simulink model "kundur_cvs_v3_discrete"  (R2025b)
settings: Solver=FixedStepAuto  StartTime=0.0  StopTime=0.5  FixedStep=50e-6  RelTol=1e-3
values from neighbouring files (symbols this model uses):
  delta0_1 = 0.294539737007    [kundur_cvs_v3_discrete_runtime.mat]    (also in kundur_cvs_v3_runtime.mat)
  delta0_2 = 0.0944024626245    [kundur_cvs_v3_discrete_runtime.mat]    (also in kundur_cvs_v3_runtime.mat)
  delta0_3 = 0.25103283995    [kundur_cvs_v3_discrete_runtime.mat]    (also in kundur_cvs_v3_runtime.mat)
  delta0_4 = 0.0812572055811    [kundur_cvs_v3_discrete_runtime.mat]    (also in kundur_cvs_v3_runtime.mat)
  deltaG0_1 = 0.522124293082    [kundur_cvs_v3_discrete_runtime.mat]    (also in kundur_cvs_v3_runtime.mat)
  deltaG0_2 = 0.476153951225    [kundur_cvs_v3_discrete_runtime.mat]    (also in kundur_cvs_v3_runtime.mat)
  deltaG0_3 = 0.293879837027    [kundur_cvs_v3_discrete_runtime.mat]    (also in kundur_cvs_v3_runtime.mat)
  Dg_1 = 5    [kundur_cvs_v3_discrete_runtime.mat]    (also in kundur_cvs_v3_runtime.mat)
  Dg_2 = 5    [kundur_cvs_v3_discrete_runtime.mat]    (also in kundur_cvs_v3_runtime.mat)
  Dg_3 = 5    [kundur_cvs_v3_discrete_runtime.mat]    (also in kundur_cvs_v3_runtime.mat)
  LoadStep_amp_bus14 = 248000000    [kundur_cvs_v3_discrete_runtime.mat]    (also in kundur_cvs_v3_runtime.mat)
  LoadStep_amp_bus15 = 0    [kundur_cvs_v3_discrete_runtime.mat]    (also in kundur_cvs_v3_runtime.mat)
  LoadStep_t_bus14 = 5    [kundur_cvs_v3_discrete_runtime.mat]    (also in kundur_cvs_v3_runtime.mat)
  LoadStep_t_bus15 = 5    [kundur_cvs_v3_discrete_runtime.mat]    (also in kundur_cvs_v3_runtime.mat)
  Mg_1 = 13    [kundur_cvs_v3_discrete_runtime.mat]    (also in kundur_cvs_v3_runtime.mat)
  Mg_2 = 13    [kundur_cvs_v3_discrete_runtime.mat]    (also in kundur_cvs_v3_runtime.mat)
  Mg_3 = 12.35    [kundur_cvs_v3_discrete_runtime.mat]    (also in kundur_cvs_v3_runtime.mat)
  Pe_scale = 1e-08    [kundur_cvs_runtime.mat]    (also in kundur_cvs_v3_discrete_runtime.mat; kundur_cvs_v3_runtime.mat)
  Pm_1 = 0.250224865012    [kundur_cvs_v3_discrete_runtime.mat]    (also in kundur_cvs_v3_runtime.mat)
  Pm_2 = 0.250224865012    [kundur_cvs_v3_discrete_runtime.mat]    (also in kundur_cvs_v3_runtime.mat)
  Pm_3 = 0.250224865012    [kundur_cvs_v3_discrete_runtime.mat]    (also in kundur_cvs_v3_runtime.mat)
  Pm_4 = 0.250224865012    [kundur_cvs_v3_discrete_runtime.mat]    (also in kundur_cvs_v3_runtime.mat)
  Pmg_1 = 7.00000000011    [kundur_cvs_v3_discrete_runtime.mat]    (also in kundur_cvs_v3_runtime.mat)
  Pmg_2 = 7    [kundur_cvs_v3_discrete_runtime.mat]    (also in kundur_cvs_v3_runtime.mat)
  Pmg_3 = 7.19    [kundur_cvs_v3_discrete_runtime.mat]    (also in kundur_cvs_v3_runtime.mat)
  PmgStep_amp_1 = 0    [kundur_cvs_v3_discrete_runtime.mat]    (also in kundur_cvs_v3_runtime.mat)
  PmgStep_amp_2 = 0    [kundur_cvs_v3_discrete_runtime.mat]    (also in kundur_cvs_v3_runtime.mat)
  PmgStep_amp_3 = 0    [kundur_cvs_v3_discrete_runtime.mat]    (also in kundur_cvs_v3_runtime.mat)
  PmgStep_t_1 = 5    [kundur_cvs_v3_discrete_runtime.mat]    (also in kundur_cvs_v3_runtime.mat)
  PmgStep_t_2 = 5    [kundur_cvs_v3_discrete_runtime.mat]    (also in kundur_cvs_v3_runtime.mat)
  PmgStep_t_3 = 5    [kundur_cvs_v3_discrete_runtime.mat]    (also in kundur_cvs_v3_runtime.mat)
  Rg_1 = 0.05    [kundur_cvs_v3_discrete_runtime.mat]    (also in kundur_cvs_v3_runtime.mat)
  Rg_2 = 0.05    [kundur_cvs_v3_discrete_runtime.mat]    (also in kundur_cvs_v3_runtime.mat)
  Rg_3 = 0.05    [kundur_cvs_v3_discrete_runtime.mat]    (also in kundur_cvs_v3_runtime.mat)
  SGScale_1 = 0.111111111111    [kundur_cvs_v3_discrete_runtime.mat]    (also in kundur_cvs_v3_runtime.mat)
  SGScale_2 = 0.111111111111    [kundur_cvs_v3_discrete_runtime.mat]    (also in kundur_cvs_v3_runtime.mat)
  SGScale_3 = 0.111111111111    [kundur_cvs_v3_discrete_runtime.mat]    (also in kundur_cvs_v3_runtime.mat)
  VemfG_1 = 266775.927939    [kundur_cvs_v3_discrete_runtime.mat]    (also in kundur_cvs_v3_runtime.mat)
  VemfG_2 = 255963.649879    [kundur_cvs_v3_discrete_runtime.mat]    (also in kundur_cvs_v3_runtime.mat)
  VemfG_3 = 266432.593136    [kundur_cvs_v3_discrete_runtime.mat]    (also in kundur_cvs_v3_runtime.mat)
  Vmag_1 = 230000    [kundur_cvs_runtime.mat]    (also in kundur_cvs_v3_discrete_runtime.mat = 201813.659575; kundur_cvs_v3_runtime.mat = 201813.659575)
  Vmag_2 = 230000    [kundur_cvs_runtime.mat]    (also in kundur_cvs_v3_discrete_runtime.mat = 232642.850172; kundur_cvs_v3_runtime.mat = 232642.850172)
  Vmag_3 = 230000    [kundur_cvs_runtime.mat]    (also in kundur_cvs_v3_discrete_runtime.mat = 178957.562058; kundur_cvs_v3_runtime.mat = 178957.562058)
  Vmag_4 = 230000    [kundur_cvs_runtime.mat]    (also in kundur_cvs_v3_discrete_runtime.mat = 226974.072481; kundur_cvs_v3_runtime.mat = 226974.072481)
  VSGScale_1 = 0.5    [kundur_cvs_v3_discrete_runtime.mat]    (also in kundur_cvs_v3_runtime.mat)
  VSGScale_2 = 0.5    [kundur_cvs_v3_discrete_runtime.mat]    (also in kundur_cvs_v3_runtime.mat)
  VSGScale_3 = 0.5    [kundur_cvs_v3_discrete_runtime.mat]    (also in kundur_cvs_v3_runtime.mat)
  VSGScale_4 = 0.5    [kundur_cvs_v3_discrete_runtime.mat]    (also in kundur_cvs_v3_runtime.mat)
  WindAmp_1 = 1    [kundur_cvs_v3_discrete_runtime.mat]    (also in kundur_cvs_v3_runtime.mat)
  WindAmp_2 = 1    [kundur_cvs_v3_discrete_runtime.mat]    (also in kundur_cvs_v3_runtime.mat)
  wn_const = 314.159265359    [kundur_cvs_runtime.mat]    (also in kundur_cvs_v3_discrete_runtime.mat; kundur_cvs_v3_runtime.mat)
  Wphase_1 = 0.0648179941055    [kundur_cvs_v3_discrete_runtime.mat]    (also in kundur_cvs_v3_runtime.mat)
  Wphase_2 = 0.0587091014116    [kundur_cvs_v3_discrete_runtime.mat]    (also in kundur_cvs_v3_runtime.mat)
  WVmag_1 = 230000    [kundur_cvs_v3_discrete_runtime.mat]    (also in kundur_cvs_v3_runtime.mat)
  WVmag_2 = 230000    [kundur_cvs_v3_discrete_runtime.mat]    (also in kundur_cvs_v3_runtime.mat)
undefined symbols (not defined in the file or in its folder): D_1, D_2, D_3, D_4, M_1, M_2, M_3, M_4, Pm_step_amp_1, Pm_step_amp_2, Pm_step_amp_3, Pm_step_amp_4, Pm_step_t_1, Pm_step_t_2, Pm_step_t_3, Pm_step_t_4
libraries: spsControlledVoltageSourceLib x21, spsSeriesRLCBranchLib x21, spsThreePhasePISectionLineLib x19, spsGroundLib x7, spsThreePhaseVIMeasurementLib x7, spsThreePhaseSeriesRLCLoadLib x6, spsThreePhaseBreakerLib x2, spsThreePhaseSourceLib x2, spspowerguiLib x1
settings Model: Creator=27443  LastModifiedBy=27443

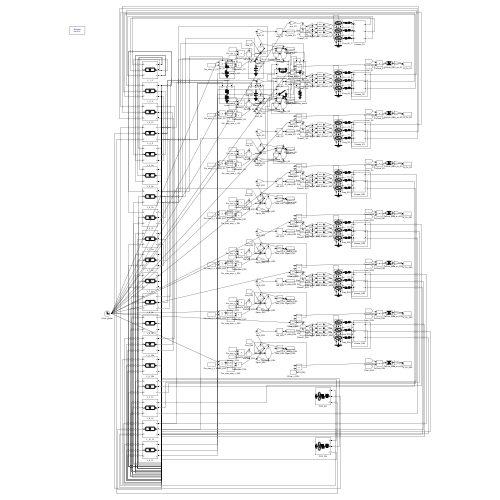
[thumbnail: Simulink's stored preview of the top-level diagram]
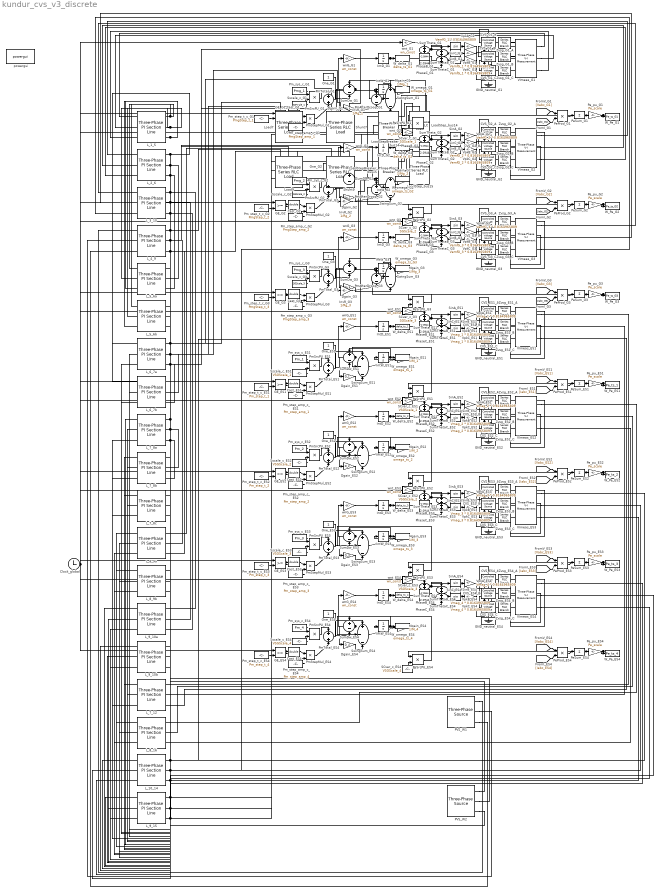
== system kundur_cvs_v3_discrete ==
  CVS_ES1_A : spsControlledVoltageSourceLib/Controlled Voltage Source  Initialize=on  Source_Type=AC  Amplitude=0  Phase=0  Frequency=0  Measurements=None
  CVS_ES1_B : spsControlledVoltageSourceLib/Controlled Voltage Source  Initialize=on  Source_Type=AC  Amplitude=0  Phase=0  Frequency=0  Measurements=None
  CVS_ES1_C : spsControlledVoltageSourceLib/Controlled Voltage Source  Initialize=on  Source_Type=AC  Amplitude=0  Phase=0  Frequency=0  Measurements=None
  CVS_ES2_A : spsControlledVoltageSourceLib/Controlled Voltage Source  Initialize=on  Source_Type=AC  Amplitude=0  Phase=0  Frequency=0  Measurements=None
  CVS_ES2_B : spsControlledVoltageSourceLib/Controlled Voltage Source  Initialize=on  Source_Type=AC  Amplitude=0  Phase=0  Frequency=0  Measurements=None
  CVS_ES2_C : spsControlledVoltageSourceLib/Controlled Voltage Source  Initialize=on  Source_Type=AC  Amplitude=0  Phase=0  Frequency=0  Measurements=None
  CVS_ES3_A : spsControlledVoltageSourceLib/Controlled Voltage Source  Initialize=on  Source_Type=AC  Amplitude=0  Phase=0  Frequency=0  Measurements=None
  CVS_ES3_B : spsControlledVoltageSourceLib/Controlled Voltage Source  Initialize=on  Source_Type=AC  Amplitude=0  Phase=0  Frequency=0  Measurements=None
  CVS_ES3_C : spsControlledVoltageSourceLib/Controlled Voltage Source  Initialize=on  Source_Type=AC  Amplitude=0  Phase=0  Frequency=0  Measurements=None
  CVS_ES4_A : spsControlledVoltageSourceLib/Controlled Voltage Source  Initialize=on  Source_Type=AC  Amplitude=0  Phase=0  Frequency=0  Measurements=None
  CVS_ES4_B : spsControlledVoltageSourceLib/Controlled Voltage Source  Initialize=on  Source_Type=AC  Amplitude=0  Phase=0  Frequency=0  Measurements=None
  CVS_ES4_C : spsControlledVoltageSourceLib/Controlled Voltage Source  Initialize=on  Source_Type=AC  Amplitude=0  Phase=0  Frequency=0  Measurements=None
  CVS_G1_A : spsControlledVoltageSourceLib/Controlled Voltage Source  Initialize=on  Source_Type=AC  Amplitude=0  Phase=0  Frequency=0  Measurements=None
  CVS_G1_B : spsControlledVoltageSourceLib/Controlled Voltage Source  Initialize=on  Source_Type=AC  Amplitude=0  Phase=0  Frequency=0  Measurements=None
  CVS_G1_C : spsControlledVoltageSourceLib/Controlled Voltage Source  Initialize=on  Source_Type=AC  Amplitude=0  Phase=0  Frequency=0  Measurements=None
  CVS_G2_A : spsControlledVoltageSourceLib/Controlled Voltage Source  Initialize=on  Source_Type=AC  Amplitude=0  Phase=0  Frequency=0  Measurements=None
  CVS_G2_B : spsControlledVoltageSourceLib/Controlled Voltage Source  Initialize=on  Source_Type=AC  Amplitude=0  Phase=0  Frequency=0  Measurements=None
  CVS_G2_C : spsControlledVoltageSourceLib/Controlled Voltage Source  Initialize=on  Source_Type=AC  Amplitude=0  Phase=0  Frequency=0  Measurements=None
  CVS_G3_A : spsControlledVoltageSourceLib/Controlled Voltage Source  Initialize=on  Source_Type=AC  Amplitude=0  Phase=0  Frequency=0  Measurements=None
  CVS_G3_B : spsControlledVoltageSourceLib/Controlled Voltage Source  Initialize=on  Source_Type=AC  Amplitude=0  Phase=0  Frequency=0  Measurements=None
  CVS_G3_C : spsControlledVoltageSourceLib/Controlled Voltage Source  Initialize=on  Source_Type=AC  Amplitude=0  Phase=0  Frequency=0  Measurements=None
  Cast_ES{1..4} (4 alike) : DataTypeConversion  OutDataTypeStr=double  SaturateOnIntegerOverflow=off  RndMeth=Floor
  Cast_G1 : DataTypeConversion  OutDataTypeStr=double  SaturateOnIntegerOverflow=off  RndMeth=Floor
  Cast_G2 : DataTypeConversion  OutDataTypeStr=double  SaturateOnIntegerOverflow=off  RndMeth=Floor
  Cast_G3 : DataTypeConversion  OutDataTypeStr=double  SaturateOnIntegerOverflow=off  RndMeth=Floor
  Clock_global : Clock
  Dgain_ES1 : Gain  Gain=D_1
  Dgain_ES2 : Gain  Gain=D_2
  Dgain_ES3 : Gain  Gain=D_3
  Dgain_ES4 : Gain  Gain=D_4
  Dgain_G1 : Gain  Gain=Dg_1
  Dgain_G2 : Gain  Gain=Dg_2
  Dgain_G3 : Gain  Gain=Dg_3
  GE_ES{1..4} (4 alike) : RelationalOperator  OutDataTypeStr=boolean  RndMeth=Simplest  InputSameDT=off
  GE_G1 : RelationalOperator  OutDataTypeStr=boolean  RndMeth=Simplest  InputSameDT=off
  GE_G2 : RelationalOperator  OutDataTypeStr=boolean  RndMeth=Simplest  InputSameDT=off
  GE_G3 : RelationalOperator  OutDataTypeStr=boolean  RndMeth=Simplest  InputSameDT=off
  GND_neutral_ES{1..4} (4 alike) : spsGroundLib/Ground  LConnTagsString=a
  GND_neutral_G1 : spsGroundLib/Ground  LConnTagsString=a
  GND_neutral_G2 : spsGroundLib/Ground  LConnTagsString=a
  GND_neutral_G3 : spsGroundLib/Ground  LConnTagsString=a
  IntD_ES1 : Integrator  InitialCondition=delta0_1
  IntD_ES2 : Integrator  InitialCondition=delta0_2
  IntD_ES3 : Integrator  InitialCondition=delta0_3
  IntD_ES4 : Integrator  InitialCondition=delta0_4
  IntD_G1 : Integrator  InitialCondition=deltaG0_1
  IntD_G2 : Integrator  InitialCondition=deltaG0_2
  IntD_G3 : Integrator  InitialCondition=deltaG0_3
  IntW_ES{1..4} (4 alike) : Integrator  InitialCondition=1
  IntW_G1 : Integrator  InitialCondition=1
  IntW_G2 : Integrator  InitialCondition=1
  IntW_G3 : Integrator  InitialCondition=1
  InvR_G1 : Gain  Gain=1/Rg_1
  InvR_G2 : Gain  Gain=1/Rg_2
  InvR_G3 : Gain  Gain=1/Rg_3
  L_10_14 : spsThreePhasePISectionLineLib/Three-Phase PI Section Line  LConnTagsString=a|b|c  RConnTagsString=A|B|C  Length=1  Frequency=50  Resistances=[0.01 0.03]  Inductances=[0.0005 0.0015]  Capacitances=[2.55102040816327e-08 1.53061224489796e-08]
  L_1_5 : spsThreePhasePISectionLineLib/Three-Phase PI Section Line  LConnTagsString=a|b|c  RConnTagsString=A|B|C  Length=5  Frequency=50  Resistances=[0.053 0.159]  Inductances=[0.00141 0.00423]  Capacitances=[9.04617166015342e-09 5.42770299609205e-09]
  L_2_6 : spsThreePhasePISectionLineLib/Three-Phase PI Section Line  LConnTagsString=a|b|c  RConnTagsString=A|B|C  Length=5  Frequency=50  Resistances=[0.053 0.159]  Inductances=[0.00141 0.00423]  Capacitances=[9.04617166015342e-09 5.42770299609205e-09]
  L_3_10 : spsThreePhasePISectionLineLib/Three-Phase PI Section Line  LConnTagsString=a|b|c  RConnTagsString=A|B|C  Length=5  Frequency=50  Resistances=[0.053 0.159]  Inductances=[0.00141 0.00423]  Capacitances=[9.04617166015342e-09 5.42770299609205e-09]
  L_4_9 : spsThreePhasePISectionLineLib/Three-Phase PI Section Line  LConnTagsString=a|b|c  RConnTagsString=A|B|C  Length=5  Frequency=50  Resistances=[0.053 0.159]  Inductances=[0.00141 0.00423]  Capacitances=[9.04617166015342e-09 5.42770299609205e-09]
  L_5_6a : spsThreePhasePISectionLineLib/Three-Phase PI Section Line  LConnTagsString=a|b|c  RConnTagsString=A|B|C  Length=25  Frequency=50  Resistances=[0.053 0.159]  Inductances=[0.00141 0.00423]  Capacitances=[9.04617166015342e-09 5.42770299609205e-09]
  L_5_6b : spsThreePhasePISectionLineLib/Three-Phase PI Section Line  LConnTagsString=a|b|c  RConnTagsString=A|B|C  Length=25  Frequency=50  Resistances=[0.053 0.159]  Inductances=[0.00141 0.00423]  Capacitances=[9.04617166015342e-09 5.42770299609205e-09]
  L_6_7a : spsThreePhasePISectionLineLib/Three-Phase PI Section Line  LConnTagsString=a|b|c  RConnTagsString=A|B|C  Length=10  Frequency=50  Resistances=[0.053 0.159]  Inductances=[0.00141 0.00423]  Capacitances=[9.04617166015342e-09 5.42770299609205e-09]
  L_6_7b : spsThreePhasePISectionLineLib/Three-Phase PI Section Line  LConnTagsString=a|b|c  RConnTagsString=A|B|C  Length=10  Frequency=50  Resistances=[0.053 0.159]  Inductances=[0.00141 0.00423]  Capacitances=[9.04617166015342e-09 5.42770299609205e-09]
  L_7_12 : spsThreePhasePISectionLineLib/Three-Phase PI Section Line  LConnTagsString=a|b|c  RConnTagsString=A|B|C  Length=1  Frequency=50  Resistances=[0.01 0.03]  Inductances=[0.0005 0.0015]  Capacitances=[2.55102040816327e-08 1.53061224489796e-08]
  L_7_8a : spsThreePhasePISectionLineLib/Three-Phase PI Section Line  LConnTagsString=a|b|c  RConnTagsString=A|B|C  Length=110  Frequency=50  Resistances=[0.053 0.159]  Inductances=[0.00141 0.00423]  Capacitances=[9.04617166015342e-09 5.42770299609205e-09]
  L_7_8b : spsThreePhasePISectionLineLib/Three-Phase PI Section Line  LConnTagsString=a|b|c  RConnTagsString=A|B|C  Length=110  Frequency=50  Resistances=[0.053 0.159]  Inductances=[0.00141 0.00423]  Capacitances=[9.04617166015342e-09 5.42770299609205e-09]
  L_7_8c : spsThreePhasePISectionLineLib/Three-Phase PI Section Line  LConnTagsString=a|b|c  RConnTagsString=A|B|C  Length=110  Frequency=50  Resistances=[0.053 0.159]  Inductances=[0.00141 0.00423]  Capacitances=[9.04617166015342e-09 5.42770299609205e-09]
  L_8_16 : spsThreePhasePISectionLineLib/Three-Phase PI Section Line  LConnTagsString=a|b|c  RConnTagsString=A|B|C  Length=1  Frequency=50  Resistances=[0.01 0.03]  Inductances=[0.0005 0.0015]  Capacitances=[2.55102040816327e-08 1.53061224489796e-08]
  L_8_9a : spsThreePhasePISectionLineLib/Three-Phase PI Section Line  LConnTagsString=a|b|c  RConnTagsString=A|B|C  Length=10  Frequency=50  Resistances=[0.053 0.159]  Inductances=[0.00141 0.00423]  Capacitances=[9.04617166015342e-09 5.42770299609205e-09]
  L_8_9b : spsThreePhasePISectionLineLib/Three-Phase PI Section Line  LConnTagsString=a|b|c  RConnTagsString=A|B|C  Length=10  Frequency=50  Resistances=[0.053 0.159]  Inductances=[0.00141 0.00423]  Capacitances=[9.04617166015342e-09 5.42770299609205e-09]
  L_9_10a : spsThreePhasePISectionLineLib/Three-Phase PI Section Line  LConnTagsString=a|b|c  RConnTagsString=A|B|C  Length=25  Frequency=50  Resistances=[0.053 0.159]  Inductances=[0.00141 0.00423]  Capacitances=[9.04617166015342e-09 5.42770299609205e-09]
  L_9_10b : spsThreePhasePISectionLineLib/Three-Phase PI Section Line  LConnTagsString=a|b|c  RConnTagsString=A|B|C  Length=25  Frequency=50  Resistances=[0.053 0.159]  Inductances=[0.00141 0.00423]  Capacitances=[9.04617166015342e-09 5.42770299609205e-09]
  L_9_15 : spsThreePhasePISectionLineLib/Three-Phase PI Section Line  LConnTagsString=a|b|c  RConnTagsString=A|B|C  Length=1  Frequency=50  Resistances=[0.01 0.03]  Inductances=[0.0005 0.0015]  Capacitances=[2.55102040816327e-08 1.53061224489796e-08]
  Load7 : spsThreePhaseSeriesRLCLoadLib/Three-Phase Series RLC Load  LConnTagsString=A|B|C  Configuration=Y (grounded)  NominalVoltage=230000  Vabc=[1e3 1e3 1e3]  Vabcp=[1e3 1e3 1e3]  NominalFrequency=50  UnbalancedPower=off  ActivePower=967000000  InductivePower=100000000  CapacitivePower=0  Pabc=[10e3 9e3 11e3]  QLabc=[100 90 110]  QCabc=[100 90 110]  Pabcp=[10e3 9e3 11e3]  QLabcp=[100 90 110]  QCabcp=[100 90 110]  Measurements=None  LoadType=constant Z
  Load9 : spsThreePhaseSeriesRLCLoadLib/Three-Phase Series RLC Load  LConnTagsString=A|B|C  Configuration=Y (grounded)  NominalVoltage=230000  Vabc=[1e3 1e3 1e3]  Vabcp=[1e3 1e3 1e3]  NominalFrequency=50  UnbalancedPower=off  ActivePower=1767000000  InductivePower=100000000  CapacitivePower=0  Pabc=[10e3 9e3 11e3]  QLabc=[100 90 110]  QCabc=[100 90 110]  Pabcp=[10e3 9e3 11e3]  QLabcp=[100 90 110]  QCabcp=[100 90 110]  Measurements=None  LoadType=constant Z
  LoadStepBreaker_bus14 : spsThreePhaseBreakerLib/Three-Phase Breaker  InitialState=closed  SwitchA=on  SwitchB=on  SwitchC=on  SwitchTimes=[LoadStep_t_bus14]  External=off  BreakerResistance=0.01  SnubberResistance=1e6  SnubberCapacitance=inf  Measurements=None
  LoadStepBreaker_bus15 : spsThreePhaseBreakerLib/Three-Phase Breaker  InitialState=open  SwitchA=on  SwitchB=on  SwitchC=on  SwitchTimes=[LoadStep_t_bus15]  External=off  BreakerResistance=0.01  SnubberResistance=1e6  SnubberCapacitance=inf  Measurements=None
  LoadStep_bus14 : spsThreePhaseSeriesRLCLoadLib/Three-Phase Series RLC Load  LConnTagsString=A|B|C  Configuration=Y (grounded)  NominalVoltage=230000  Vabc=[1e3 1e3 1e3]  Vabcp=[1e3 1e3 1e3]  NominalFrequency=50  UnbalancedPower=off  ActivePower=max(LoadStep_amp_bus14, 1)  InductivePower=0  CapacitivePower=0  Pabc=[10e3 9e3 11e3]  QLabc=[100 90 110]  QCabc=[100 90 110]  Pabcp=[10e3 9e3 11e3]  QLabcp=[100 90 110]  QCabcp=[100 90 110]  Measurements=None  LoadType=constant Z
  LoadStep_bus15 : spsThreePhaseSeriesRLCLoadLib/Three-Phase Series RLC Load  LConnTagsString=A|B|C  Configuration=Y (grounded)  NominalVoltage=230000  Vabc=[1e3 1e3 1e3]  Vabcp=[1e3 1e3 1e3]  NominalFrequency=50  UnbalancedPower=off  ActivePower=max(LoadStep_amp_bus15, 1)  InductivePower=0  CapacitivePower=0  Pabc=[10e3 9e3 11e3]  QLabc=[100 90 110]  QCabc=[100 90 110]  Pabcp=[10e3 9e3 11e3]  QLabcp=[100 90 110]  QCabcp=[100 90 110]  Measurements=None  LoadType=constant Z
  Mgain_ES1 : Gain  Gain=1/M_1
  Mgain_ES2 : Gain  Gain=1/M_2
  Mgain_ES3 : Gain  Gain=1/M_3
  Mgain_ES4 : Gain  Gain=1/M_4
  Mgain_G1 : Gain  Gain=1/Mg_1
  Mgain_G2 : Gain  Gain=1/Mg_2
  Mgain_G3 : Gain  Gain=1/Mg_3
  One_ES{1..4} (4 alike) : Constant
  One_G1 : Constant
  One_G2 : Constant
  One_G3 : Constant
  PVS_W1 : spsThreePhaseSourceLib/Three-Phase Source  InternalConnection=Yg  VoltagePhases=off  Voltage=(WindAmp_1) * (WVmag_1)  PhaseAngle=(Wphase_1) * 180/pi  Voltage_phases=[25e3 25e3 25e3]/sqrt(3)  PhaseAngles_phases=[0 -120 +120]  Frequency=50  NonIdealSource=on  SpecifyImpedance=on  Resistance=0.8929  Inductance=16.58e-3  ShortCircuitLevel=500e6  BaseVoltage=230000  XRratio=7  BusType=swing  Pref=10e3  Qref=0  Prefabc=[10e3, 10e3, 10e3]  Qrefabc=[0, 0, 0]  Qmin=-inf  Qmax=inf
  PVS_W2 : spsThreePhaseSourceLib/Three-Phase Source  InternalConnection=Yg  VoltagePhases=off  Voltage=(WindAmp_2) * (WVmag_2)  PhaseAngle=(Wphase_2) * 180/pi  Voltage_phases=[25e3 25e3 25e3]/sqrt(3)  PhaseAngles_phases=[0 -120 +120]  Frequency=50  NonIdealSource=on  SpecifyImpedance=on  Resistance=0.8929  Inductance=16.58e-3  ShortCircuitLevel=500e6  BaseVoltage=230000  XRratio=7  BusType=swing  Pref=10e3  Qref=0  Prefabc=[10e3, 10e3, 10e3]  Qrefabc=[0, 0, 0]  Qmin=-inf  Qmax=inf
  PeProd_ES{1..4} (4 alike) : Product
  PeProd_G1 : Product
  PeProd_G2 : Product
  PeProd_G3 : Product
  PeSrcPU_ES{1..4} (4 alike) : Product
  PeSrcPU_G1 : Product
  PeSrcPU_G2 : Product
  PeSrcPU_G3 : Product
  PeSum_ES{1..4} (4 alike) : Sum  Inputs=+
  PeSum_G1 : Sum  Inputs=+
  PeSum_G2 : Sum  Inputs=+
  PeSum_G3 : Sum  Inputs=+
  Pe_pu_ES{1..4} (4 alike) : Gain  Gain=Pe_scale
  Pe_pu_G1 : Gain  Gain=Pe_scale
  Pe_pu_G2 : Gain  Gain=Pe_scale
  Pe_pu_G3 : Gain  Gain=Pe_scale
  PhaseB_ES{1..4} (4 alike) : Constant  Value=-2.0944
  PhaseB_G1 : Constant  Value=-2.0944
  PhaseB_G2 : Constant  Value=-2.0944
  PhaseB_G3 : Constant  Value=-2.0944
  PhaseC_ES{1..4} (4 alike) : Constant  Value=2.0944
  PhaseC_G1 : Constant  Value=2.0944
  PhaseC_G2 : Constant  Value=2.0944
  PhaseC_G3 : Constant  Value=2.0944
  PmAfterDroop_G1 : Sum  Inputs=+-
  PmAfterDroop_G2 : Sum  Inputs=+-
  PmAfterDroop_G3 : Sum  Inputs=+-
  PmSrcPU_ES{1..4} (4 alike) : Product
  PmSrcPU_G1 : Product
  PmSrcPU_G2 : Product
  PmSrcPU_G3 : Product
  PmStepMul_ES{1..4} (4 alike) : Product
  PmStepMul_G1 : Product
  PmStepMul_G2 : Product
  PmStepMul_G3 : Product
  PmTotal_ES{1..4} (4 alike) : Sum
  PmTotal_G1 : Sum
  PmTotal_G2 : Sum
  PmTotal_G3 : Sum
  Pm_step_amp_c_ES1 : Constant  Value=Pm_step_amp_1
  Pm_step_amp_c_ES2 : Constant  Value=Pm_step_amp_2
  Pm_step_amp_c_ES3 : Constant  Value=Pm_step_amp_3
  Pm_step_amp_c_ES4 : Constant  Value=Pm_step_amp_4
  Pm_step_amp_c_G1 : Constant  Value=PmgStep_amp_1
  Pm_step_amp_c_G2 : Constant  Value=PmgStep_amp_2
  Pm_step_amp_c_G3 : Constant  Value=PmgStep_amp_3
  Pm_step_t_c_ES1 : Constant  Value=Pm_step_t_1
  Pm_step_t_c_ES2 : Constant  Value=Pm_step_t_2
  Pm_step_t_c_ES3 : Constant  Value=Pm_step_t_3
  Pm_step_t_c_ES4 : Constant  Value=Pm_step_t_4
  Pm_step_t_c_G1 : Constant  Value=PmgStep_t_1
  Pm_step_t_c_G2 : Constant  Value=PmgStep_t_2
  Pm_step_t_c_G3 : Constant  Value=PmgStep_t_3
  Pm_sys_c_ES1 : Constant  Value=Pm_1
  Pm_sys_c_ES2 : Constant  Value=Pm_2
  Pm_sys_c_ES3 : Constant  Value=Pm_3
  Pm_sys_c_ES4 : Constant  Value=Pm_4
  Pm_sys_c_G1 : Constant  Value=Pmg_1
  Pm_sys_c_G2 : Constant  Value=Pmg_2
  Pm_sys_c_G3 : Constant  Value=Pmg_3
  SCvar_c_ES1 : Constant  Value=VSGScale_1
  SCvar_c_ES2 : Constant  Value=VSGScale_2
  SCvar_c_ES3 : Constant  Value=VSGScale_3
  SCvar_c_ES4 : Constant  Value=VSGScale_4
  SCvar_c_G1 : Constant  Value=SGScale_1
  SCvar_c_G2 : Constant  Value=SGScale_2
  SCvar_c_G3 : Constant  Value=SGScale_3
  Shunt7 : spsThreePhaseSeriesRLCLoadLib/Three-Phase Series RLC Load  LConnTagsString=A|B|C  Configuration=Y (grounded)  NominalVoltage=230000  Vabc=[1e3 1e3 1e3]  Vabcp=[1e3 1e3 1e3]  NominalFrequency=50  UnbalancedPower=off  ActivePower=0  InductivePower=0  CapacitivePower=200000000  Pabc=[10e3 9e3 11e3]  QLabc=[100 90 110]  QCabc=[100 90 110]  Pabcp=[10e3 9e3 11e3]  QLabcp=[100 90 110]  QCabcp=[100 90 110]  Measurements=None  LoadType=constant Z
  Shunt9 : spsThreePhaseSeriesRLCLoadLib/Three-Phase Series RLC Load  LConnTagsString=A|B|C  Configuration=Y (grounded)  NominalVoltage=230000  Vabc=[1e3 1e3 1e3]  Vabcp=[1e3 1e3 1e3]  NominalFrequency=50  UnbalancedPower=off  ActivePower=0  InductivePower=0  CapacitivePower=350000000  Pabc=[10e3 9e3 11e3]  QLabc=[100 90 110]  QCabc=[100 90 110]  Pabcp=[10e3 9e3 11e3]  QLabcp=[100 90 110]  QCabcp=[100 90 110]  Measurements=None  LoadType=constant Z
  SinA_ES{1..4} (4 alike) : Trigonometry
  SinA_G1 : Trigonometry
  SinA_G2 : Trigonometry
  SinA_G3 : Trigonometry
  SinB_ES{1..4} (4 alike) : Trigonometry
  SinB_G1 : Trigonometry
  SinB_G2 : Trigonometry
  SinB_G3 : Trigonometry
  SinC_ES{1..4} (4 alike) : Trigonometry
  SinC_G1 : Trigonometry
  SinC_G2 : Trigonometry
  SinC_G3 : Trigonometry
  Sscale_c_ES1 : Constant  Value=VSGScale_1
  Sscale_c_ES2 : Constant  Value=VSGScale_2
  Sscale_c_ES3 : Constant  Value=VSGScale_3
  Sscale_c_ES4 : Constant  Value=VSGScale_4
  Sscale_c_G1 : Constant  Value=SGScale_1
  Sscale_c_G2 : Constant  Value=SGScale_2
  Sscale_c_G3 : Constant  Value=SGScale_3
  SumDw_ES{1..4} (4 alike) : Sum  Inputs=+-
  SumDw_G1 : Sum  Inputs=+-
  SumDw_G2 : Sum  Inputs=+-
  SumDw_G3 : Sum  Inputs=+-
  SumThetaB_ES{1..4} (4 alike) : Sum
  SumThetaB_G1 : Sum
  SumThetaB_G2 : Sum
  SumThetaB_G3 : Sum
  SumThetaC_ES{1..4} (4 alike) : Sum
  SumThetaC_G1 : Sum
  SumThetaC_G2 : Sum
  SumThetaC_G3 : Sum
  SumTheta_ES{1..4} (4 alike) : Sum
  SumTheta_G1 : Sum
  SumTheta_G2 : Sum
  SumTheta_G3 : Sum
  SwingSum_ES{1..4} (4 alike) : Sum  Inputs=+--
  SwingSum_G1 : Sum  Inputs=+--
  SwingSum_G2 : Sum  Inputs=+--
  SwingSum_G3 : Sum  Inputs=+--
  VImeas_ES1 : spsThreePhaseVIMeasurementLib/Three-Phase V-I Measurement  VoltageMeasurement=phase-to-ground  SetLabelV=on  LabelV=Vabc_ES1  Vpu=off  VpuLL=off  CurrentMeasurement=yes  SetLabelI=on  LabelI=Iabc_ES1  Ipu=off  Pbase=100e6  Vbase=500e3  OutputType=Complex  PhasorSimulation=off  PSBequivalent=0
  VImeas_ES2 : spsThreePhaseVIMeasurementLib/Three-Phase V-I Measurement  VoltageMeasurement=phase-to-ground  SetLabelV=on  LabelV=Vabc_ES2  Vpu=off  VpuLL=off  CurrentMeasurement=yes  SetLabelI=on  LabelI=Iabc_ES2  Ipu=off  Pbase=100e6  Vbase=500e3  OutputType=Complex  PhasorSimulation=off  PSBequivalent=0
  VImeas_ES3 : spsThreePhaseVIMeasurementLib/Three-Phase V-I Measurement  VoltageMeasurement=phase-to-ground  SetLabelV=on  LabelV=Vabc_ES3  Vpu=off  VpuLL=off  CurrentMeasurement=yes  SetLabelI=on  LabelI=Iabc_ES3  Ipu=off  Pbase=100e6  Vbase=500e3  OutputType=Complex  PhasorSimulation=off  PSBequivalent=0
  VImeas_ES4 : spsThreePhaseVIMeasurementLib/Three-Phase V-I Measurement  VoltageMeasurement=phase-to-ground  SetLabelV=on  LabelV=Vabc_ES4  Vpu=off  VpuLL=off  CurrentMeasurement=yes  SetLabelI=on  LabelI=Iabc_ES4  Ipu=off  Pbase=100e6  Vbase=500e3  OutputType=Complex  PhasorSimulation=off  PSBequivalent=0
  VImeas_G1 : spsThreePhaseVIMeasurementLib/Three-Phase V-I Measurement  VoltageMeasurement=phase-to-ground  SetLabelV=on  LabelV=Vabc_G1  Vpu=off  VpuLL=off  CurrentMeasurement=yes  SetLabelI=on  LabelI=Iabc_G1  Ipu=off  Pbase=100e6  Vbase=500e3  OutputType=Complex  PhasorSimulation=off  PSBequivalent=0
  VImeas_G2 : spsThreePhaseVIMeasurementLib/Three-Phase V-I Measurement  VoltageMeasurement=phase-to-ground  SetLabelV=on  LabelV=Vabc_G2  Vpu=off  VpuLL=off  CurrentMeasurement=yes  SetLabelI=on  LabelI=Iabc_G2  Ipu=off  Pbase=100e6  Vbase=500e3  OutputType=Complex  PhasorSimulation=off  PSBequivalent=0
  VImeas_G3 : spsThreePhaseVIMeasurementLib/Three-Phase V-I Measurement  VoltageMeasurement=phase-to-ground  SetLabelV=on  LabelV=Vabc_G3  Vpu=off  VpuLL=off  CurrentMeasurement=yes  SetLabelI=on  LabelI=Iabc_G3  Ipu=off  Pbase=100e6  Vbase=500e3  OutputType=Complex  PhasorSimulation=off  PSBequivalent=0
  VpkA_ES1 : Gain  Gain=Vmag_1 * 0.8164965809
  VpkA_ES2 : Gain  Gain=Vmag_2 * 0.8164965809
  VpkA_ES3 : Gain  Gain=Vmag_3 * 0.8164965809
  VpkA_ES4 : Gain  Gain=Vmag_4 * 0.8164965809
  VpkA_G1 : Gain  Gain=VemfG_1 * 0.8164965809
  VpkA_G2 : Gain  Gain=VemfG_2 * 0.8164965809
  VpkA_G3 : Gain  Gain=VemfG_3 * 0.8164965809
  VpkB_ES1 : Gain  Gain=Vmag_1 * 0.8164965809
  VpkB_ES2 : Gain  Gain=Vmag_2 * 0.8164965809
  VpkB_ES3 : Gain  Gain=Vmag_3 * 0.8164965809
  VpkB_ES4 : Gain  Gain=Vmag_4 * 0.8164965809
  VpkB_G1 : Gain  Gain=VemfG_1 * 0.8164965809
  VpkB_G2 : Gain  Gain=VemfG_2 * 0.8164965809
  VpkB_G3 : Gain  Gain=VemfG_3 * 0.8164965809
  VpkC_ES1 : Gain  Gain=Vmag_1 * 0.8164965809
  VpkC_ES2 : Gain  Gain=Vmag_2 * 0.8164965809
  VpkC_ES3 : Gain  Gain=Vmag_3 * 0.8164965809
  VpkC_ES4 : Gain  Gain=Vmag_4 * 0.8164965809
  VpkC_G1 : Gain  Gain=VemfG_1 * 0.8164965809
  VpkC_G2 : Gain  Gain=VemfG_2 * 0.8164965809
  VpkC_G3 : Gain  Gain=VemfG_3 * 0.8164965809
  W_Pe_ES1 : ToWorkspace  VariableName=Pe_ts_1  SaveFormat=Timeseries  SampleTime=-1
      settings: MaxDataPoints=2
  W_Pe_ES2 : ToWorkspace  VariableName=Pe_ts_2  SaveFormat=Timeseries  SampleTime=-1
      settings: MaxDataPoints=2
  W_Pe_ES3 : ToWorkspace  VariableName=Pe_ts_3  SaveFormat=Timeseries  SampleTime=-1
      settings: MaxDataPoints=2
  W_Pe_ES4 : ToWorkspace  VariableName=Pe_ts_4  SaveFormat=Timeseries  SampleTime=-1
      settings: MaxDataPoints=2
  W_Pe_G1 : ToWorkspace  VariableName=Pe_ts_G1  SaveFormat=Timeseries  SampleTime=-1
      settings: MaxDataPoints=2
  W_Pe_G2 : ToWorkspace  VariableName=Pe_ts_G2  SaveFormat=Timeseries  SampleTime=-1
      settings: MaxDataPoints=2
  W_Pe_G3 : ToWorkspace  VariableName=Pe_ts_G3  SaveFormat=Timeseries  SampleTime=-1
      settings: MaxDataPoints=2
  W_delta_ES1 : ToWorkspace  VariableName=delta_ts_1  SaveFormat=Timeseries  SampleTime=-1
      settings: MaxDataPoints=2
  W_delta_ES2 : ToWorkspace  VariableName=delta_ts_2  SaveFormat=Timeseries  SampleTime=-1
      settings: MaxDataPoints=2
  W_delta_ES3 : ToWorkspace  VariableName=delta_ts_3  SaveFormat=Timeseries  SampleTime=-1
      settings: MaxDataPoints=2
  W_delta_ES4 : ToWorkspace  VariableName=delta_ts_4  SaveFormat=Timeseries  SampleTime=-1
      settings: MaxDataPoints=2
  W_delta_G1 : ToWorkspace  VariableName=delta_ts_G1  SaveFormat=Timeseries  SampleTime=-1
      settings: MaxDataPoints=2
  W_delta_G2 : ToWorkspace  VariableName=delta_ts_G2  SaveFormat=Timeseries  SampleTime=-1
      settings: MaxDataPoints=2
  W_delta_G3 : ToWorkspace  VariableName=delta_ts_G3  SaveFormat=Timeseries  SampleTime=-1
      settings: MaxDataPoints=2
  W_omega_ES1 : ToWorkspace  VariableName=omega_ts_1  SaveFormat=Timeseries  SampleTime=-1
      settings: MaxDataPoints=2
  W_omega_ES2 : ToWorkspace  VariableName=omega_ts_2  SaveFormat=Timeseries  SampleTime=-1
      settings: MaxDataPoints=2
  W_omega_ES3 : ToWorkspace  VariableName=omega_ts_3  SaveFormat=Timeseries  SampleTime=-1
      settings: MaxDataPoints=2
  W_omega_ES4 : ToWorkspace  VariableName=omega_ts_4  SaveFormat=Timeseries  SampleTime=-1
      settings: MaxDataPoints=2
  W_omega_G1 : ToWorkspace  VariableName=omega_ts_G1  SaveFormat=Timeseries  SampleTime=-1
      settings: MaxDataPoints=2
  W_omega_G2 : ToWorkspace  VariableName=omega_ts_G2  SaveFormat=Timeseries  SampleTime=-1
      settings: MaxDataPoints=2
  W_omega_G3 : ToWorkspace  VariableName=omega_ts_G3  SaveFormat=Timeseries  SampleTime=-1
      settings: MaxDataPoints=2
  Zvsg_ES1_A : spsSeriesRLCBranchLib/Series RLC Branch  LConnTagsString=__new0  RConnTagsString=__new0  BranchType=RL  Resistance=0.7935  Inductance=0.25258  SetiL0=off  InitialCurrent=0  Capacitance=1e-6  Setx0=off  InitialVoltage=0  Measurements=None
  Zvsg_ES1_B : spsSeriesRLCBranchLib/Series RLC Branch  LConnTagsString=__new0  RConnTagsString=__new0  BranchType=RL  Resistance=0.7935  Inductance=0.25258  SetiL0=off  InitialCurrent=0  Capacitance=1e-6  Setx0=off  InitialVoltage=0  Measurements=None
  Zvsg_ES1_C : spsSeriesRLCBranchLib/Series RLC Branch  LConnTagsString=__new0  RConnTagsString=__new0  BranchType=RL  Resistance=0.7935  Inductance=0.25258  SetiL0=off  InitialCurrent=0  Capacitance=1e-6  Setx0=off  InitialVoltage=0  Measurements=None
  Zvsg_ES2_A : spsSeriesRLCBranchLib/Series RLC Branch  LConnTagsString=__new0  RConnTagsString=__new0  BranchType=RL  Resistance=0.7935  Inductance=0.25258  SetiL0=off  InitialCurrent=0  Capacitance=1e-6  Setx0=off  InitialVoltage=0  Measurements=None
  Zvsg_ES2_B : spsSeriesRLCBranchLib/Series RLC Branch  LConnTagsString=__new0  RConnTagsString=__new0  BranchType=RL  Resistance=0.7935  Inductance=0.25258  SetiL0=off  InitialCurrent=0  Capacitance=1e-6  Setx0=off  InitialVoltage=0  Measurements=None
  Zvsg_ES2_C : spsSeriesRLCBranchLib/Series RLC Branch  LConnTagsString=__new0  RConnTagsString=__new0  BranchType=RL  Resistance=0.7935  Inductance=0.25258  SetiL0=off  InitialCurrent=0  Capacitance=1e-6  Setx0=off  InitialVoltage=0  Measurements=None
  Zvsg_ES3_A : spsSeriesRLCBranchLib/Series RLC Branch  LConnTagsString=__new0  RConnTagsString=__new0  BranchType=RL  Resistance=0.7935  Inductance=0.25258  SetiL0=off  InitialCurrent=0  Capacitance=1e-6  Setx0=off  InitialVoltage=0  Measurements=None
  Zvsg_ES3_B : spsSeriesRLCBranchLib/Series RLC Branch  LConnTagsString=__new0  RConnTagsString=__new0  BranchType=RL  Resistance=0.7935  Inductance=0.25258  SetiL0=off  InitialCurrent=0  Capacitance=1e-6  Setx0=off  InitialVoltage=0  Measurements=None
  Zvsg_ES3_C : spsSeriesRLCBranchLib/Series RLC Branch  LConnTagsString=__new0  RConnTagsString=__new0  BranchType=RL  Resistance=0.7935  Inductance=0.25258  SetiL0=off  InitialCurrent=0  Capacitance=1e-6  Setx0=off  InitialVoltage=0  Measurements=None
  Zvsg_ES4_A : spsSeriesRLCBranchLib/Series RLC Branch  LConnTagsString=__new0  RConnTagsString=__new0  BranchType=RL  Resistance=0.7935  Inductance=0.25258  SetiL0=off  InitialCurrent=0  Capacitance=1e-6  Setx0=off  InitialVoltage=0  Measurements=None
  Zvsg_ES4_B : spsSeriesRLCBranchLib/Series RLC Branch  LConnTagsString=__new0  RConnTagsString=__new0  BranchType=RL  Resistance=0.7935  Inductance=0.25258  SetiL0=off  InitialCurrent=0  Capacitance=1e-6  Setx0=off  InitialVoltage=0  Measurements=None
  Zvsg_ES4_C : spsSeriesRLCBranchLib/Series RLC Branch  LConnTagsString=__new0  RConnTagsString=__new0  BranchType=RL  Resistance=0.7935  Inductance=0.25258  SetiL0=off  InitialCurrent=0  Capacitance=1e-6  Setx0=off  InitialVoltage=0  Measurements=None
  Zvsg_G1_A : spsSeriesRLCBranchLib/Series RLC Branch  LConnTagsString=__new0  RConnTagsString=__new0  BranchType=RL  Resistance=0.7935  Inductance=0.056129  SetiL0=off  InitialCurrent=0  Capacitance=1e-6  Setx0=off  InitialVoltage=0  Measurements=None
  Zvsg_G1_B : spsSeriesRLCBranchLib/Series RLC Branch  LConnTagsString=__new0  RConnTagsString=__new0  BranchType=RL  Resistance=0.7935  Inductance=0.056129  SetiL0=off  InitialCurrent=0  Capacitance=1e-6  Setx0=off  InitialVoltage=0  Measurements=None
  Zvsg_G1_C : spsSeriesRLCBranchLib/Series RLC Branch  LConnTagsString=__new0  RConnTagsString=__new0  BranchType=RL  Resistance=0.7935  Inductance=0.056129  SetiL0=off  InitialCurrent=0  Capacitance=1e-6  Setx0=off  InitialVoltage=0  Measurements=None
  Zvsg_G2_A : spsSeriesRLCBranchLib/Series RLC Branch  LConnTagsString=__new0  RConnTagsString=__new0  BranchType=RL  Resistance=0.7935  Inductance=0.056129  SetiL0=off  InitialCurrent=0  Capacitance=1e-6  Setx0=off  InitialVoltage=0  Measurements=None
  Zvsg_G2_B : spsSeriesRLCBranchLib/Series RLC Branch  LConnTagsString=__new0  RConnTagsString=__new0  BranchType=RL  Resistance=0.7935  Inductance=0.056129  SetiL0=off  InitialCurrent=0  Capacitance=1e-6  Setx0=off  InitialVoltage=0  Measurements=None
  Zvsg_G2_C : spsSeriesRLCBranchLib/Series RLC Branch  LConnTagsString=__new0  RConnTagsString=__new0  BranchType=RL  Resistance=0.7935  Inductance=0.056129  SetiL0=off  InitialCurrent=0  Capacitance=1e-6  Setx0=off  InitialVoltage=0  Measurements=None
  Zvsg_G3_A : spsSeriesRLCBranchLib/Series RLC Branch  LConnTagsString=__new0  RConnTagsString=__new0  BranchType=RL  Resistance=0.7935  Inductance=0.056129  SetiL0=off  InitialCurrent=0  Capacitance=1e-6  Setx0=off  InitialVoltage=0  Measurements=None
  Zvsg_G3_B : spsSeriesRLCBranchLib/Series RLC Branch  LConnTagsString=__new0  RConnTagsString=__new0  BranchType=RL  Resistance=0.7935  Inductance=0.056129  SetiL0=off  InitialCurrent=0  Capacitance=1e-6  Setx0=off  InitialVoltage=0  Measurements=None
  Zvsg_G3_C : spsSeriesRLCBranchLib/Series RLC Branch  LConnTagsString=__new0  RConnTagsString=__new0  BranchType=RL  Resistance=0.7935  Inductance=0.056129  SetiL0=off  InitialCurrent=0  Capacitance=1e-6  Setx0=off  InitialVoltage=0  Measurements=None
  powergui : spspowerguiLib/powergui  Priority=1  SimulationMode=Discrete  SampleTime=50e-6  frequency=60  Iterations=50  frequencyindice=60  Pbase=100e6  ErrMax=1e-4  UnitsV=kV  UnitsW=MW  buscounter=0  FunctionMessages=off  echomessages=off  EnableUseOfTLC=off  CurrentSourceSwitches=off  DisableSnubberDevices=off  DisableRonSwitches=off  DisableVfSwitches=off  DisplayEquations=off  AutomaticDiscreteSolvers=off  SolverType=Tustin/Backward Euler (TBE)  Interpol=off  ExternalGateDelay=off  methode=off  Ts=100  x0status=blocks  SPID=on  SwTol=0  HookPort=off  NonlinearTolerance=1e-4  nMaxIteration=100  ContinueOnMaxIteration=off  RestoreLinks=warning  ResistiveCurrentMeasurement=off  Frange=[0:2:500]  Ylog=off  Xlog=on  ShowGrid=off  save=off  variable=ZData  structure=0  ZoomFFT=off  StartTime=0.0  cycles=1  DisplayStyle=1  fundamental=60  FreqAxis=off  MaxFrequency=1000  frequencyindicesteady=1  RmsSteady=1  display=off
  wnG_ES{1..4} (4 alike) : Gain  Gain=wn_const
  wnG_G1 : Gain  Gain=wn_const
  wnG_G2 : Gain  Gain=wn_const
  wnG_G3 : Gain  Gain=wn_const
  wnt_ES{1..4} (4 alike) : Gain  Gain=wn_const
  wnt_G1 : Gain  Gain=wn_const
  wnt_G2 : Gain  Gain=wn_const
  wnt_G3 : Gain  Gain=wn_const
  wires:
  Clock_global/1 -> GE_G1/1, wnt_G1/1, GE_G2/1, wnt_G2/1, GE_G3/1, wnt_G3/1, GE_ES1/1, wnt_ES1/1, GE_ES2/1, wnt_ES2/1, GE_ES3/1, wnt_ES3/1, GE_ES4/1, wnt_ES4/1
  Pm_step_t_c_G1/1 -> GE_G1/2
  GE_G1/1 -> Cast_G1/1
  Cast_G1/1 -> PmStepMul_G1/1
  Pm_step_amp_c_G1/1 -> PmStepMul_G1/2
  Pm_sys_c_G1/1 -> PmSrcPU_G1/1
  Sscale_c_G1/1 -> PmSrcPU_G1/2
  PmSrcPU_G1/1 -> PmTotal_G1/1
  PmStepMul_G1/1 -> PmTotal_G1/2
  IntW_G1/1 -> SumDw_G1/1, W_omega_G1/1
  One_G1/1 -> SumDw_G1/2
  SumDw_G1/1 -> Dgain_G1/1, InvR_G1/1, wnG_G1/1
  PmTotal_G1/1 -> PmAfterDroop_G1/1
  InvR_G1/1 -> PmAfterDroop_G1/2
  PmAfterDroop_G1/1 -> SwingSum_G1/1
  Dgain_G1/1 -> SwingSum_G1/3
  SwingSum_G1/1 -> Mgain_G1/1
  Mgain_G1/1 -> IntW_G1/1
  wnG_G1/1 -> IntD_G1/1
  wnt_G1/1 -> SumTheta_G1/1
  IntD_G1/1 -> SumTheta_G1/2, W_delta_G1/1
  SumTheta_G1/1 -> SumThetaB_G1/1, SumThetaC_G1/1, SinA_G1/1
  PhaseB_G1/1 -> SumThetaB_G1/2
  PhaseC_G1/1 -> SumThetaC_G1/2
  SumThetaB_G1/1 -> SinB_G1/1
  SumThetaC_G1/1 -> SinC_G1/1
  SinA_G1/1 -> VpkA_G1/1
  SinB_G1/1 -> VpkB_G1/1
  SinC_G1/1 -> VpkC_G1/1
  VpkA_G1/1 -> CVS_G1_A/1
  VpkB_G1/1 -> CVS_G1_B/1
  VpkC_G1/1 -> CVS_G1_C/1
  [Vabc_G1] -> PeProd_G1/1
  [Iabc_G1] -> PeProd_G1/2
  PeProd_G1/1 -> PeSum_G1/1
  PeSum_G1/1 -> Pe_pu_G1/1
  Pe_pu_G1/1 -> PeSrcPU_G1/1, W_Pe_G1/1
  SCvar_c_G1/1 -> PeSrcPU_G1/2
  PeSrcPU_G1/1 -> SwingSum_G1/2
  Pm_step_t_c_G2/1 -> GE_G2/2
  GE_G2/1 -> Cast_G2/1
  Cast_G2/1 -> PmStepMul_G2/1
  Pm_step_amp_c_G2/1 -> PmStepMul_G2/2
  Pm_sys_c_G2/1 -> PmSrcPU_G2/1
  Sscale_c_G2/1 -> PmSrcPU_G2/2
  PmSrcPU_G2/1 -> PmTotal_G2/1
  PmStepMul_G2/1 -> PmTotal_G2/2
  IntW_G2/1 -> SumDw_G2/1, W_omega_G2/1
  One_G2/1 -> SumDw_G2/2
  SumDw_G2/1 -> Dgain_G2/1, InvR_G2/1, wnG_G2/1
  PmTotal_G2/1 -> PmAfterDroop_G2/1
  InvR_G2/1 -> PmAfterDroop_G2/2
  PmAfterDroop_G2/1 -> SwingSum_G2/1
  Dgain_G2/1 -> SwingSum_G2/3
  SwingSum_G2/1 -> Mgain_G2/1
  Mgain_G2/1 -> IntW_G2/1
  wnG_G2/1 -> IntD_G2/1
  wnt_G2/1 -> SumTheta_G2/1
  IntD_G2/1 -> SumTheta_G2/2, W_delta_G2/1
  SumTheta_G2/1 -> SumThetaB_G2/1, SumThetaC_G2/1, SinA_G2/1
  PhaseB_G2/1 -> SumThetaB_G2/2
  PhaseC_G2/1 -> SumThetaC_G2/2
  SumThetaB_G2/1 -> SinB_G2/1
  SumThetaC_G2/1 -> SinC_G2/1
  SinA_G2/1 -> VpkA_G2/1
  SinB_G2/1 -> VpkB_G2/1
  SinC_G2/1 -> VpkC_G2/1
  VpkA_G2/1 -> CVS_G2_A/1
  VpkB_G2/1 -> CVS_G2_B/1
  VpkC_G2/1 -> CVS_G2_C/1
  [Vabc_G2] -> PeProd_G2/1
  [Iabc_G2] -> PeProd_G2/2
  PeProd_G2/1 -> PeSum_G2/1
  PeSum_G2/1 -> Pe_pu_G2/1
  Pe_pu_G2/1 -> PeSrcPU_G2/1, W_Pe_G2/1
  SCvar_c_G2/1 -> PeSrcPU_G2/2
  PeSrcPU_G2/1 -> SwingSum_G2/2
  Pm_step_t_c_G3/1 -> GE_G3/2
  GE_G3/1 -> Cast_G3/1
  Cast_G3/1 -> PmStepMul_G3/1
  Pm_step_amp_c_G3/1 -> PmStepMul_G3/2
  Pm_sys_c_G3/1 -> PmSrcPU_G3/1
  Sscale_c_G3/1 -> PmSrcPU_G3/2
  PmSrcPU_G3/1 -> PmTotal_G3/1
  PmStepMul_G3/1 -> PmTotal_G3/2
  IntW_G3/1 -> SumDw_G3/1, W_omega_G3/1
  One_G3/1 -> SumDw_G3/2
  SumDw_G3/1 -> Dgain_G3/1, InvR_G3/1, wnG_G3/1
  PmTotal_G3/1 -> PmAfterDroop_G3/1
  InvR_G3/1 -> PmAfterDroop_G3/2
  PmAfterDroop_G3/1 -> SwingSum_G3/1
  Dgain_G3/1 -> SwingSum_G3/3
  SwingSum_G3/1 -> Mgain_G3/1
  Mgain_G3/1 -> IntW_G3/1
  wnG_G3/1 -> IntD_G3/1
  wnt_G3/1 -> SumTheta_G3/1
  IntD_G3/1 -> SumTheta_G3/2, W_delta_G3/1
  SumTheta_G3/1 -> SumThetaB_G3/1, SumThetaC_G3/1, SinA_G3/1
  PhaseB_G3/1 -> SumThetaB_G3/2
  PhaseC_G3/1 -> SumThetaC_G3/2
  SumThetaB_G3/1 -> SinB_G3/1
  SumThetaC_G3/1 -> SinC_G3/1
  SinA_G3/1 -> VpkA_G3/1
  SinB_G3/1 -> VpkB_G3/1
  SinC_G3/1 -> VpkC_G3/1
  VpkA_G3/1 -> CVS_G3_A/1
  VpkB_G3/1 -> CVS_G3_B/1
  VpkC_G3/1 -> CVS_G3_C/1
  [Vabc_G3] -> PeProd_G3/1
  [Iabc_G3] -> PeProd_G3/2
  PeProd_G3/1 -> PeSum_G3/1
  PeSum_G3/1 -> Pe_pu_G3/1
  Pe_pu_G3/1 -> PeSrcPU_G3/1, W_Pe_G3/1
  SCvar_c_G3/1 -> PeSrcPU_G3/2
  PeSrcPU_G3/1 -> SwingSum_G3/2
  Pm_step_t_c_ES1/1 -> GE_ES1/2
  GE_ES1/1 -> Cast_ES1/1
  Cast_ES1/1 -> PmStepMul_ES1/1
  Pm_step_amp_c_ES1/1 -> PmStepMul_ES1/2
  Pm_sys_c_ES1/1 -> PmSrcPU_ES1/1
  Sscale_c_ES1/1 -> PmSrcPU_ES1/2
  PmSrcPU_ES1/1 -> PmTotal_ES1/1
  PmStepMul_ES1/1 -> PmTotal_ES1/2
  IntW_ES1/1 -> SumDw_ES1/1, W_omega_ES1/1
  One_ES1/1 -> SumDw_ES1/2
  SumDw_ES1/1 -> Dgain_ES1/1, wnG_ES1/1
  PmTotal_ES1/1 -> SwingSum_ES1/1
  Dgain_ES1/1 -> SwingSum_ES1/3
  SwingSum_ES1/1 -> Mgain_ES1/1
  Mgain_ES1/1 -> IntW_ES1/1
  wnG_ES1/1 -> IntD_ES1/1
  wnt_ES1/1 -> SumTheta_ES1/1
  IntD_ES1/1 -> SumTheta_ES1/2, W_delta_ES1/1
  SumTheta_ES1/1 -> SumThetaB_ES1/1, SumThetaC_ES1/1, SinA_ES1/1
  PhaseB_ES1/1 -> SumThetaB_ES1/2
  PhaseC_ES1/1 -> SumThetaC_ES1/2
  SumThetaB_ES1/1 -> SinB_ES1/1
  SumThetaC_ES1/1 -> SinC_ES1/1
  SinA_ES1/1 -> VpkA_ES1/1
  SinB_ES1/1 -> VpkB_ES1/1
  SinC_ES1/1 -> VpkC_ES1/1
  VpkA_ES1/1 -> CVS_ES1_A/1
  VpkB_ES1/1 -> CVS_ES1_B/1
  VpkC_ES1/1 -> CVS_ES1_C/1
  [Vabc_ES1] -> PeProd_ES1/1
  [Iabc_ES1] -> PeProd_ES1/2
  PeProd_ES1/1 -> PeSum_ES1/1
  PeSum_ES1/1 -> Pe_pu_ES1/1
  Pe_pu_ES1/1 -> PeSrcPU_ES1/1, W_Pe_ES1/1
  SCvar_c_ES1/1 -> PeSrcPU_ES1/2
  PeSrcPU_ES1/1 -> SwingSum_ES1/2
  Pm_step_t_c_ES2/1 -> GE_ES2/2
  GE_ES2/1 -> Cast_ES2/1
  Cast_ES2/1 -> PmStepMul_ES2/1
  Pm_step_amp_c_ES2/1 -> PmStepMul_ES2/2
  Pm_sys_c_ES2/1 -> PmSrcPU_ES2/1
  Sscale_c_ES2/1 -> PmSrcPU_ES2/2
  PmSrcPU_ES2/1 -> PmTotal_ES2/1
  PmStepMul_ES2/1 -> PmTotal_ES2/2
  IntW_ES2/1 -> SumDw_ES2/1, W_omega_ES2/1
  One_ES2/1 -> SumDw_ES2/2
  SumDw_ES2/1 -> Dgain_ES2/1, wnG_ES2/1
  PmTotal_ES2/1 -> SwingSum_ES2/1
  Dgain_ES2/1 -> SwingSum_ES2/3
  SwingSum_ES2/1 -> Mgain_ES2/1
  Mgain_ES2/1 -> IntW_ES2/1
  wnG_ES2/1 -> IntD_ES2/1
  wnt_ES2/1 -> SumTheta_ES2/1
  IntD_ES2/1 -> SumTheta_ES2/2, W_delta_ES2/1
  SumTheta_ES2/1 -> SumThetaB_ES2/1, SumThetaC_ES2/1, SinA_ES2/1
  PhaseB_ES2/1 -> SumThetaB_ES2/2
  PhaseC_ES2/1 -> SumThetaC_ES2/2
  SumThetaB_ES2/1 -> SinB_ES2/1
  SumThetaC_ES2/1 -> SinC_ES2/1
  SinA_ES2/1 -> VpkA_ES2/1
  SinB_ES2/1 -> VpkB_ES2/1
  SinC_ES2/1 -> VpkC_ES2/1
  VpkA_ES2/1 -> CVS_ES2_A/1
  VpkB_ES2/1 -> CVS_ES2_B/1
  VpkC_ES2/1 -> CVS_ES2_C/1
  [Vabc_ES2] -> PeProd_ES2/1
  [Iabc_ES2] -> PeProd_ES2/2
  PeProd_ES2/1 -> PeSum_ES2/1
  PeSum_ES2/1 -> Pe_pu_ES2/1
  Pe_pu_ES2/1 -> PeSrcPU_ES2/1, W_Pe_ES2/1
  SCvar_c_ES2/1 -> PeSrcPU_ES2/2
  PeSrcPU_ES2/1 -> SwingSum_ES2/2
  Pm_step_t_c_ES3/1 -> GE_ES3/2
  GE_ES3/1 -> Cast_ES3/1
  Cast_ES3/1 -> PmStepMul_ES3/1
  Pm_step_amp_c_ES3/1 -> PmStepMul_ES3/2
  Pm_sys_c_ES3/1 -> PmSrcPU_ES3/1
  Sscale_c_ES3/1 -> PmSrcPU_ES3/2
  PmSrcPU_ES3/1 -> PmTotal_ES3/1
  PmStepMul_ES3/1 -> PmTotal_ES3/2
  IntW_ES3/1 -> SumDw_ES3/1, W_omega_ES3/1
  One_ES3/1 -> SumDw_ES3/2
  SumDw_ES3/1 -> Dgain_ES3/1, wnG_ES3/1
  PmTotal_ES3/1 -> SwingSum_ES3/1
  Dgain_ES3/1 -> SwingSum_ES3/3
  SwingSum_ES3/1 -> Mgain_ES3/1
  Mgain_ES3/1 -> IntW_ES3/1
  wnG_ES3/1 -> IntD_ES3/1
  wnt_ES3/1 -> SumTheta_ES3/1
  IntD_ES3/1 -> SumTheta_ES3/2, W_delta_ES3/1
  SumTheta_ES3/1 -> SumThetaB_ES3/1, SumThetaC_ES3/1, SinA_ES3/1
  PhaseB_ES3/1 -> SumThetaB_ES3/2
  PhaseC_ES3/1 -> SumThetaC_ES3/2
  SumThetaB_ES3/1 -> SinB_ES3/1
  SumThetaC_ES3/1 -> SinC_ES3/1
  SinA_ES3/1 -> VpkA_ES3/1
  SinB_ES3/1 -> VpkB_ES3/1
  SinC_ES3/1 -> VpkC_ES3/1
  VpkA_ES3/1 -> CVS_ES3_A/1
  VpkB_ES3/1 -> CVS_ES3_B/1
  VpkC_ES3/1 -> CVS_ES3_C/1
  [Vabc_ES3] -> PeProd_ES3/1
  [Iabc_ES3] -> PeProd_ES3/2
  PeProd_ES3/1 -> PeSum_ES3/1
  PeSum_ES3/1 -> Pe_pu_ES3/1
  Pe_pu_ES3/1 -> PeSrcPU_ES3/1, W_Pe_ES3/1
  SCvar_c_ES3/1 -> PeSrcPU_ES3/2
  PeSrcPU_ES3/1 -> SwingSum_ES3/2
  Pm_step_t_c_ES4/1 -> GE_ES4/2
  GE_ES4/1 -> Cast_ES4/1
  Cast_ES4/1 -> PmStepMul_ES4/1
  Pm_step_amp_c_ES4/1 -> PmStepMul_ES4/2
  Pm_sys_c_ES4/1 -> PmSrcPU_ES4/1
  Sscale_c_ES4/1 -> PmSrcPU_ES4/2
  PmSrcPU_ES4/1 -> PmTotal_ES4/1
  PmStepMul_ES4/1 -> PmTotal_ES4/2
  IntW_ES4/1 -> SumDw_ES4/1, W_omega_ES4/1
  One_ES4/1 -> SumDw_ES4/2
  SumDw_ES4/1 -> Dgain_ES4/1, wnG_ES4/1
  PmTotal_ES4/1 -> SwingSum_ES4/1
  Dgain_ES4/1 -> SwingSum_ES4/3
  SwingSum_ES4/1 -> Mgain_ES4/1
  Mgain_ES4/1 -> IntW_ES4/1
  wnG_ES4/1 -> IntD_ES4/1
  wnt_ES4/1 -> SumTheta_ES4/1
  IntD_ES4/1 -> SumTheta_ES4/2, W_delta_ES4/1
  SumTheta_ES4/1 -> SumThetaB_ES4/1, SumThetaC_ES4/1, SinA_ES4/1
  PhaseB_ES4/1 -> SumThetaB_ES4/2
  PhaseC_ES4/1 -> SumThetaC_ES4/2
  SumThetaB_ES4/1 -> SinB_ES4/1
  SumThetaC_ES4/1 -> SinC_ES4/1
  SinA_ES4/1 -> VpkA_ES4/1
  SinB_ES4/1 -> VpkB_ES4/1
  SinC_ES4/1 -> VpkC_ES4/1
  VpkA_ES4/1 -> CVS_ES4_A/1
  VpkB_ES4/1 -> CVS_ES4_B/1
  VpkC_ES4/1 -> CVS_ES4_C/1
  [Vabc_ES4] -> PeProd_ES4/1
  [Iabc_ES4] -> PeProd_ES4/2
  PeProd_ES4/1 -> PeSum_ES4/1
  PeSum_ES4/1 -> Pe_pu_ES4/1
  Pe_pu_ES4/1 -> PeSrcPU_ES4/1, W_Pe_ES4/1
  SCvar_c_ES4/1 -> PeSrcPU_ES4/2
  PeSrcPU_ES4/1 -> SwingSum_ES4/2
  connections:
  LoadStepBreaker_bus14/RConn1 -- LoadStep_bus14/LConn1
  LoadStepBreaker_bus14/RConn2 -- LoadStep_bus14/LConn2
  LoadStepBreaker_bus14/RConn3 -- LoadStep_bus14/LConn3
  LoadStepBreaker_bus15/RConn1 -- LoadStep_bus15/LConn1
  LoadStepBreaker_bus15/RConn2 -- LoadStep_bus15/LConn2
  LoadStepBreaker_bus15/RConn3 -- LoadStep_bus15/LConn3
  CVS_G1_A/LConn1 -- CVS_G1_B/LConn1 -- GND_neutral_G1/LConn1 -- CVS_G1_C/LConn1
  CVS_G1_A/RConn1 -- Zvsg_G1_A/LConn1
  CVS_G1_B/RConn1 -- Zvsg_G1_B/LConn1
  CVS_G1_C/RConn1 -- Zvsg_G1_C/LConn1
  Zvsg_G1_A/RConn1 -- VImeas_G1/LConn1
  Zvsg_G1_B/RConn1 -- VImeas_G1/LConn2
  Zvsg_G1_C/RConn1 -- VImeas_G1/LConn3
  CVS_G2_A/LConn1 -- CVS_G2_B/LConn1 -- GND_neutral_G2/LConn1 -- CVS_G2_C/LConn1
  CVS_G2_A/RConn1 -- Zvsg_G2_A/LConn1
  CVS_G2_B/RConn1 -- Zvsg_G2_B/LConn1
  CVS_G2_C/RConn1 -- Zvsg_G2_C/LConn1
  Zvsg_G2_A/RConn1 -- VImeas_G2/LConn1
  Zvsg_G2_B/RConn1 -- VImeas_G2/LConn2
  Zvsg_G2_C/RConn1 -- VImeas_G2/LConn3
  CVS_G3_A/LConn1 -- CVS_G3_B/LConn1 -- GND_neutral_G3/LConn1 -- CVS_G3_C/LConn1
  CVS_G3_A/RConn1 -- Zvsg_G3_A/LConn1
  CVS_G3_B/RConn1 -- Zvsg_G3_B/LConn1
  CVS_G3_C/RConn1 -- Zvsg_G3_C/LConn1
  Zvsg_G3_A/RConn1 -- VImeas_G3/LConn1
  Zvsg_G3_B/RConn1 -- VImeas_G3/LConn2
  Zvsg_G3_C/RConn1 -- VImeas_G3/LConn3
  CVS_ES1_A/LConn1 -- CVS_ES1_B/LConn1 -- GND_neutral_ES1/LConn1 -- CVS_ES1_C/LConn1
  CVS_ES1_A/RConn1 -- Zvsg_ES1_A/LConn1
  CVS_ES1_B/RConn1 -- Zvsg_ES1_B/LConn1
  CVS_ES1_C/RConn1 -- Zvsg_ES1_C/LConn1
  Zvsg_ES1_A/RConn1 -- VImeas_ES1/LConn1
  Zvsg_ES1_B/RConn1 -- VImeas_ES1/LConn2
  Zvsg_ES1_C/RConn1 -- VImeas_ES1/LConn3
  CVS_ES2_A/LConn1 -- CVS_ES2_B/LConn1 -- GND_neutral_ES2/LConn1 -- CVS_ES2_C/LConn1
  CVS_ES2_A/RConn1 -- Zvsg_ES2_A/LConn1
  CVS_ES2_B/RConn1 -- Zvsg_ES2_B/LConn1
  CVS_ES2_C/RConn1 -- Zvsg_ES2_C/LConn1
  Zvsg_ES2_A/RConn1 -- VImeas_ES2/LConn1
  Zvsg_ES2_B/RConn1 -- VImeas_ES2/LConn2
  Zvsg_ES2_C/RConn1 -- VImeas_ES2/LConn3
  CVS_ES3_A/LConn1 -- CVS_ES3_B/LConn1 -- GND_neutral_ES3/LConn1 -- CVS_ES3_C/LConn1
  CVS_ES3_A/RConn1 -- Zvsg_ES3_A/LConn1
  CVS_ES3_B/RConn1 -- Zvsg_ES3_B/LConn1
  CVS_ES3_C/RConn1 -- Zvsg_ES3_C/LConn1
  Zvsg_ES3_A/RConn1 -- VImeas_ES3/LConn1
  Zvsg_ES3_B/RConn1 -- VImeas_ES3/LConn2
  Zvsg_ES3_C/RConn1 -- VImeas_ES3/LConn3
  CVS_ES4_A/LConn1 -- CVS_ES4_B/LConn1 -- GND_neutral_ES4/LConn1 -- CVS_ES4_C/LConn1
  CVS_ES4_A/RConn1 -- Zvsg_ES4_A/LConn1
  CVS_ES4_B/RConn1 -- Zvsg_ES4_B/LConn1
  CVS_ES4_C/RConn1 -- Zvsg_ES4_C/LConn1
  Zvsg_ES4_A/RConn1 -- VImeas_ES4/LConn1
  Zvsg_ES4_B/RConn1 -- VImeas_ES4/LConn2
  Zvsg_ES4_C/RConn1 -- VImeas_ES4/LConn3
  L_1_5/RConn1 -- L_5_6a/LConn1 -- L_5_6b/LConn1
  L_1_5/RConn2 -- L_5_6a/LConn2 -- L_5_6b/LConn2
  L_1_5/RConn3 -- L_5_6a/LConn3 -- L_5_6b/LConn3
  L_5_6a/RConn1 -- L_5_6b/RConn1 -- L_6_7a/LConn1 -- L_2_6/RConn1 -- L_6_7b/LConn1
  L_5_6a/RConn2 -- L_5_6b/RConn2 -- L_6_7a/LConn2 -- L_2_6/RConn2 -- L_6_7b/LConn2
  L_5_6a/RConn3 -- L_5_6b/RConn3 -- L_6_7a/LConn3 -- L_2_6/RConn3 -- L_6_7b/LConn3
  L_6_7b/RConn1 -- L_7_8a/LConn1 -- L_7_8b/LConn1 -- L_7_8c/LConn1 -- L_7_12/LConn1 -- Load7/LConn1 -- L_6_7a/RConn1 -- Shunt7/LConn1
  L_6_7b/RConn2 -- L_7_8a/LConn2 -- L_7_8b/LConn2 -- L_7_8c/LConn2 -- L_7_12/LConn2 -- Load7/LConn2 -- L_6_7a/RConn2 -- Shunt7/LConn2
  L_6_7b/RConn3 -- L_7_8a/LConn3 -- L_7_8b/LConn3 -- L_7_8c/LConn3 -- L_7_12/LConn3 -- Load7/LConn3 -- L_6_7a/RConn3 -- Shunt7/LConn3
  L_7_8b/RConn1 -- L_7_8c/RConn1 -- L_8_9a/LConn1 -- L_8_9b/LConn1 -- L_8_16/LConn1 -- L_7_8a/RConn1 -- PVS_W2/RConn1
  L_7_8b/RConn2 -- L_7_8c/RConn2 -- L_8_9a/LConn2 -- L_8_9b/LConn2 -- L_8_16/LConn2 -- L_7_8a/RConn2 -- PVS_W2/RConn2
  L_7_8b/RConn3 -- L_7_8c/RConn3 -- L_8_9a/LConn3 -- L_8_9b/LConn3 -- L_8_16/LConn3 -- L_7_8a/RConn3 -- PVS_W2/RConn3
  L_8_9a/RConn1 -- L_8_9b/RConn1 -- L_9_10a/LConn1 -- L_9_10b/LConn1 -- L_9_15/LConn1 -- Load9/LConn1 -- L_4_9/RConn1 -- Shunt9/LConn1
  L_8_9a/RConn2 -- L_8_9b/RConn2 -- L_9_10a/LConn2 -- L_9_10b/LConn2 -- L_9_15/LConn2 -- Load9/LConn2 -- L_4_9/RConn2 -- Shunt9/LConn2
  L_8_9a/RConn3 -- L_8_9b/RConn3 -- L_9_10a/LConn3 -- L_9_10b/LConn3 -- L_9_15/LConn3 -- Load9/LConn3 -- L_4_9/RConn3 -- Shunt9/LConn3
  L_9_10a/RConn1 -- L_9_10b/RConn1 -- L_3_10/RConn1 -- L_10_14/LConn1
  L_9_10a/RConn2 -- L_9_10b/RConn2 -- L_3_10/RConn2 -- L_10_14/LConn2
  L_9_10a/RConn3 -- L_9_10b/RConn3 -- L_3_10/RConn3 -- L_10_14/LConn3
  L_10_14/RConn1 -- LoadStepBreaker_bus14/LConn1 -- VImeas_ES3/RConn1
  L_10_14/RConn2 -- LoadStepBreaker_bus14/LConn2 -- VImeas_ES3/RConn2
  L_10_14/RConn3 -- LoadStepBreaker_bus14/LConn3 -- VImeas_ES3/RConn3
  L_9_15/RConn1 -- LoadStepBreaker_bus15/LConn1 -- VImeas_ES4/RConn1
  L_9_15/RConn2 -- LoadStepBreaker_bus15/LConn2 -- VImeas_ES4/RConn2
  L_9_15/RConn3 -- LoadStepBreaker_bus15/LConn3 -- VImeas_ES4/RConn3
  VImeas_G1/RConn1 -- L_1_5/LConn1
  VImeas_G1/RConn2 -- L_1_5/LConn2
  VImeas_G1/RConn3 -- L_1_5/LConn3
  VImeas_G2/RConn1 -- L_2_6/LConn1
  VImeas_G2/RConn2 -- L_2_6/LConn2
  VImeas_G2/RConn3 -- L_2_6/LConn3
  VImeas_G3/RConn1 -- L_3_10/LConn1
  VImeas_G3/RConn2 -- L_3_10/LConn2
  VImeas_G3/RConn3 -- L_3_10/LConn3
  VImeas_ES1/RConn1 -- L_7_12/RConn1
  VImeas_ES1/RConn2 -- L_7_12/RConn2
  VImeas_ES1/RConn3 -- L_7_12/RConn3
  VImeas_ES2/RConn1 -- L_8_16/RConn1
  VImeas_ES2/RConn2 -- L_8_16/RConn2
  VImeas_ES2/RConn3 -- L_8_16/RConn3
  PVS_W1/RConn1 -- L_4_9/LConn1
  PVS_W1/RConn2 -- L_4_9/LConn2
  PVS_W1/RConn3 -- L_4_9/LConn3
